simulink model "CoVeh_TrqLeadCoord"  (R2016b)
settings: configuration reference "CodeGenConfigSet" (kept outside this file)
settings Model: Creator=wolf  LastModifiedBy=Wollf
settings ConfigSetRef: SourceLocation=Base Workspace

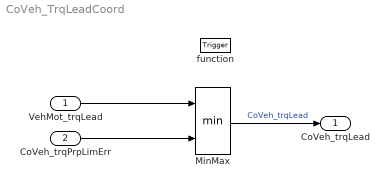
== system CoVeh_TrqLeadCoord ==
  VehMot_trqLead : Inport  Tag=Nm  Description=Lead torque for propulsion (transmission output torque)  OutMin=-3000  OutMax=3000  OutDataTypeStr=Trq_Nm
  CoVeh_trqPrpLimErr : Inport  Tag=Nm  Description=limitation torque for propulsion at system error  Port=2  OutMin=-3000  OutMax=3000  OutDataTypeStr=Trq_Nm
  function : TriggerPort  TriggerType=function-call  VariantControl=Variant
  MinMax : MinMax  Inputs=2
  CoVeh_trqLead : Outport  Tag=Nm  Description=Lead torque order on the drive train (gearbox output torque)  OutMin=-3000  OutMax=3000  OutDataTypeStr=Trq_Nm
  wires:
  VehMot_trqLead/1 -> MinMax/1
  CoVeh_trqPrpLimErr/1 -> MinMax/2
  MinMax/1 -> CoVeh_trqLead/1  "CoVeh_trqLead"
